simulink library "cdsGps"  (Simulink 6.6)
settings Model: Creator=aivanov  LastModifiedBy=aivanov  ExtModeAutoUpdateStatusClock=off

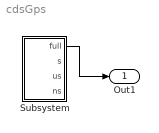
== system cdsGps ==
  Subsystem : Subsystem
  Out1 : Outport
  wires:
  Subsystem/1(full) -> Out1/1

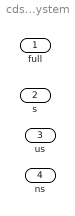
== system cdsGps/Subsystem ==
  full : Outport
  s : Outport  Port=2
  us : Outport  Port=3
  ns : Outport  Port=4
